simulink library "Fuzzy_Type2_Lib"  (R2015b)
settings: Solver=ode45  StartTime=0.0  StopTime=10.0  RelTol=1e-3
undefined symbols (not defined in the file or in its folder): evalt2
settings Model: Creator=u11f99  LastModifiedBy=Home
settings DataIOCC: SaveFormat=Array
settings OptimizationCC: ExpressionDepthLimit=2147483647
settings DebuggingCC: UnderspecifiedInitializationDetection=Classic  MergeDetectMultiDrivingBlocksExec=none  SolverPrmCheckMsg=warning  StateNameClashWarn=warning
settings HardwareCC: ProdBitPerPointer=32  ProdLargestAtomicFloat=None  ProdIntDivRoundTo=Undefined  ProdEndianess=Unspecified  ProdWordSize=32  ProdHWDeviceType=32-bit Generic
settings GRTTargetCC: GeneratePreprocessorConditionals=Disable all
settings ConfigComp: CovModelRefEnable=Off

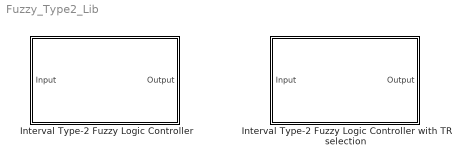
== system Fuzzy_Type2_Lib ==
  Interval Type-2 Fuzzy Logic Controller : Subsystem  mask(Type-2 Fuzzy Logic Controller){t2fisSim=0}
      mask prompts: t2fisSim "t2fis name in Workspace or File Name"
      mask Display: image(imread('MemberShipMask.jpg'))
  Interval Type-2 Fuzzy Logic Controller with TR selection : Subsystem  mask(Type-2 Fuzzy Logic Controller){t2fisSim=0, TRtype=0}
      mask prompts: t2fisSim "t2fis name in Workspace or File Name"; TRtype "Select TR method"
      mask help:
      | TR Method List for selection;
      |
      | 1 - Karnik-Mendel Algorithm (KM)
      | 2 - Enhanced Karnik-Mendel Algorithm(EKM)
      | 3 - Iterative Algorithm with Stop Condition(IASC)
      | 4 - Enhanced Iterative Algorithm with Stop Condition(EIASC)
      | 5 - Enhanced Opposite Direction Searching Algorithm(EODS)
      | 6 - wu-Mendel Uncertainity Bound Method(WM)
      | 7 - Nie-Tan Method(NT)
      | 8 - Begain-Melek-Mendel Method(BMM)
      | 9 - User Defined Function
      mask Display: image(imread('MemberShipMask.jpg'))

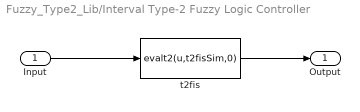
== system Fuzzy_Type2_Lib/Interval Type-2 Fuzzy Logic Controller ==
  Input : Inport
  t2fis : MATLABFcn  MATLABFcn=evalt2(u,t2fisSim,0)
  Output : Outport
  wires:
  Input/1 -> t2fis/1
  t2fis/1 -> Output/1

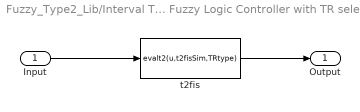
== system Fuzzy_Type2_Lib/Interval Type-2 Fuzzy Logic Controller with TR selection ==
  Input : Inport
  t2fis : MATLABFcn  MATLABFcn=evalt2(u,t2fisSim,TRtype)
  Output : Outport
  wires:
  t2fis/1 -> Output/1
  Input/1 -> t2fis/1
